simulink model "RedCraneMbsModel"  (R2024b)
settings: Solver=FixedStepAuto  StartTime=0.0  StopTime=1  FixedStep=0.001  MaxStep=0.005  RelTol=1e-3
undefined symbols (not defined in the file): thetaList0, X, Y, Z
libraries: sm_lib x75, fl_lib x18, nesl_utility x12
(part 1 of 2)
settings Model: Creator=sindr  LastModifiedBy=hagen
settings RTWCC: GPUComputeCapability=3.5
settings ConfigComp: PLC_OutputDir=plc_export\FB_InverceKinematics  PLC_TargetIDE=twincat3  PLC_MultiTBSigbuilderTimeRange=off  PLC_FoldFBCallOutputVar=off  PLC_RemoveUnusedSSMethodCallArguments=off  PLC_UseCallOutputArgSyntax=off  PLC_EnableUnsignedAndDoubleTypes=off  PLC_EnableUDTSplitting=off  PLC_MaxFieldsInUDT=500  PLC_InlineEnumCastFunction=off

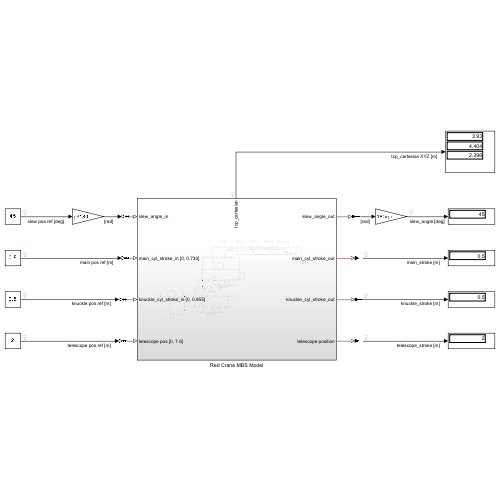
[thumbnail: Simulink's stored preview of the top-level diagram]
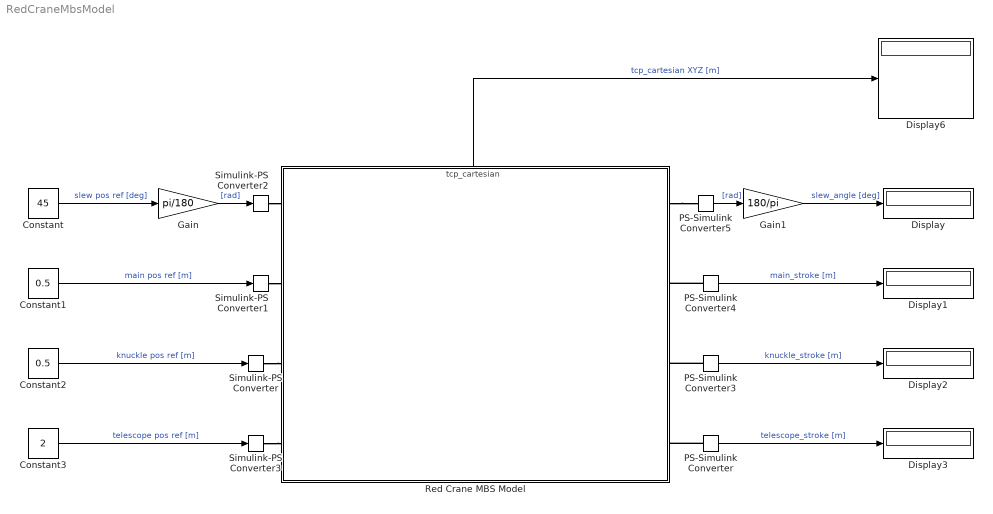
== system RedCraneMbsModel ==
  Constant : Constant  Value=45
  Constant1 : Constant  Value=0.5
  Constant2 : Constant  Value=0.5
  Constant3 : Constant  Value=2
  Display{,1..3,6} (5 alike) : Display
  Gain : Gain  Gain=pi/180
  Gain1 : Gain  Gain=180/pi
  PS-Simulink Converter{,3..5} (4 alike) : nesl_utility/PS-Simulink Converter  PhysicalDomain=network_engine_domain  SubClassName=ps_output  LeftPortType=input  RightPortType=output  PseudoPeriodic=off  Frequencies=[]  VectorFormat=inherit  Unit=inherit  AffineConversion=off
  Red Crane MBS Model : Subsystem
      settings: PortSchema="{\"entries\":[{\"content\":{\"sides\":[{\"content\":{\"connectorIds\":[\"LConn1\",\"LConn2\",\"LConn3\",\"LConn4\"]},\"type\":\"ConnectorPlacement.EquallySpacedRectSide\",\"uuid\":\"4a665765-5f1a-426d-91c2-f3af20fe3627\"},{\"content\":{\"connectorIds\":[\"RConn1\",\"RConn2\",\"RConn3\",\"RConn4\"],\"side\":\"RIGHT\"},\"type\":\"ConnectorPlacement.EquallySpacedRectSide\",\"uuid\":\"cf43645c-9a50-4bc9-b355-f38e72b1430d\"},{\"content\":{\"connectorIds\":[\"Out1\"],\"side\":\"TOP\"},\"type\":\"ConnectorPlacement.EquallySpacedRectSide\",\"uuid\":\"253dbb23-7a12-4bfe-bf07-7d8403188f09\"}]},\"type\":\"ConnectorPlacement.EquallySpacedConnector\",\"uuid\":\"5ffb1dcc-76b9-4b5c-ba8f-4653fe2f07c9\"}],\"packageUris\":[\"http://schema.mathworks.com/mf0/Connector/R2020b\"],\"version\":\"1.0\"}"
  Simulink-PS Converter{,1..3} (4 alike) : nesl_utility/Simulink-PS Converter  PhysicalDomain=network_engine_domain  SubClassName=ps_input  LeftPortType=input  RightPortType=output  PseudoPeriodic=off  Frequencies=[]  NoiseDistribution=none  NoiseParameters=[]  Unit=1  AffineConversion=off  FilteringAndDerivatives=filter  SimscapeFilterOrder=2  InputFilterTimeConstant=0.001  UdotUserProvided=0
  wires:
  PS-Simulink Converter5/1 -> Gain1/1  "[rad]"
  PS-Simulink Converter4/1 -> Display1/1  "main_stroke [m]"
  PS-Simulink Converter3/1 -> Display2/1  "knuckle_stroke [m]"
  PS-Simulink Converter/1 -> Display3/1  "telescope_stroke [m]"
  Constant/1 -> Gain/1  "slew pos ref [deg]"
  Constant1/1 -> Simulink-PS Converter1/1  "main pos ref [m]"
  Constant2/1 -> Simulink-PS Converter/1  "knuckle pos ref [m]"
  Constant3/1 -> Simulink-PS Converter3/1  "telescope pos ref [m]"
  Red Crane MBS Model/1(tcp_cartesian) -> Display6/1  "tcp_cartesian XYZ [m]"
  Gain/1 -> Simulink-PS Converter2/1  "[rad]"
  Gain1/1 -> Display/1  "slew_angle [deg]"
  connections:
  Simulink-PS Converter/RConn1 -- Red Crane MBS Model/LConn3
  Simulink-PS Converter2/RConn1 -- Red Crane MBS Model/LConn1
  Simulink-PS Converter1/RConn1 -- Red Crane MBS Model/LConn2
  Simulink-PS Converter3/RConn1 -- Red Crane MBS Model/LConn4
  PS-Simulink Converter/LConn1 -- Red Crane MBS Model/RConn4
  PS-Simulink Converter3/LConn1 -- Red Crane MBS Model/RConn3
  PS-Simulink Converter4/LConn1 -- Red Crane MBS Model/RConn2
  Red Crane MBS Model/RConn1 -- PS-Simulink Converter5/LConn1
